simulink model "directMRACSystemModel"  (Simulink 7.3)
settings: Solver=ode45  StartTime=0.0  StopTime=tf  RelTol=1e-3
InitFcn:
  | initDirectMRACSystemModel
StopFcn:
  | plotlab
values from neighbouring files (symbols this model uses):
  Am = A - b*kx'    [initDirectMRACSystemMode_wPrj.m]    (also in initDirectMRACSystemModel.m; initDirectMRACSystemModel_wStatePred.m; initL1AdaptiveSystemModel.m)
  b = [0 ; d0]    [initDirectMRACSystemMode_wPrj.m]    (also in initDirectMRACSystemModel.m; initDirectMRACSystemModel_wStatePred.m; initL1AdaptiveSystemModel.m)
  c = [1 ; 1]    [initDirectMRACSystemMode_wPrj.m]    (also in initDirectMRACSystemModel.m; initDirectMRACSystemModel_wStatePred.m; initL1AdaptiveSystemModel.m)
  fx_p_absx1x2_1 = [theta(4) 0]    [initDirectMRACSystemMode_wPrj.m]    (also in initDirectMRACSystemModel.m; initDirectMRACSystemModel_wStatePred.m; initL1AdaptiveSystemModel.m)
  fx_p_absx1x2_2 = [theta(4) 0]    [initDirectMRACSystemMode_wPrj.m]    (also in initDirectMRACSystemModel.m; initDirectMRACSystemModel_wStatePred.m; initL1AdaptiveSystemModel.m)
  fx_p_absx2x2_1 = [theta(5) 0]    [initDirectMRACSystemMode_wPrj.m]    (also in initDirectMRACSystemModel.m; initDirectMRACSystemModel_wStatePred.m; initL1AdaptiveSystemModel.m)
  fx_p_absx2x2_2 = [theta(5) 0]    [initDirectMRACSystemMode_wPrj.m]    (also in initDirectMRACSystemModel.m; initDirectMRACSystemModel_wStatePred.m; initL1AdaptiveSystemModel.m)
  fx_p_x1_1 = [theta(6) 0 theta(2) theta(1)]    [initDirectMRACSystemMode_wPrj.m]    (also in initDirectMRACSystemModel.m; initDirectMRACSystemModel_wStatePred.m; initL1AdaptiveSystemModel.m)
  fx_p_x1_2 = [theta(6) 0 theta(2) theta(1)]    [initDirectMRACSystemMode_wPrj.m]    (also in initDirectMRACSystemModel.m; initDirectMRACSystemModel_wStatePred.m; initL1AdaptiveSystemModel.m)
  fx_p_x2_1 = [theta(3) 0]    [initDirectMRACSystemMode_wPrj.m]    (also in initDirectMRACSystemModel.m; initDirectMRACSystemModel_wStatePred.m; initL1AdaptiveSystemModel.m)
  fx_p_x2_2 = [theta(3) 0]    [initDirectMRACSystemMode_wPrj.m]    (also in initDirectMRACSystemModel.m; initDirectMRACSystemModel_wStatePred.m; initL1AdaptiveSystemModel.m)
  Gamma = 1*eye(2,2)    [initDirectMRACSystemModel.m]    (also in initDirectMRACSystemModel_wStatePred.m; initL1AdaptiveSystemModel.m = 20)
  kg = -(c'*(Am^-1)*b).^-1    [initDirectMRACSystemModel.m]    (also in initDirectMRACSystemModel_wStatePred.m; initL1AdaptiveSystemModel.m)
  kx = [0.25 ; 0.707]    [initDirectMRACSystemMode_wPrj.m]    (also in initDirectMRACSystemModel.m; initDirectMRACSystemModel_wStatePred.m; initL1AdaptiveSystemModel.m)
  kxtld0 = [200 200]'    [initDirectMRACSystemMode_wPrj.m]    (also in initDirectMRACSystemModel.m = zeros(2,1))
  P = lyap(Am',Q)    [initDirectMRACSystemMode_wPrj.m]    (also in initDirectMRACSystemModel.m; initDirectMRACSystemModel_wStatePred.m; initL1AdaptiveSystemModel.m)
  tNonlinChange = tNonlinEnable+10    (= 60)    [initDirectMRACSystemMode_wPrj.m]    (also in initDirectMRACSystemModel.m = 10; initDirectMRACSystemModel_wStatePred.m = 10; initL1AdaptiveSystemModel.m = 10)
  tNonlinEnable = 50    [initDirectMRACSystemMode_wPrj.m]    (also in initDirectMRACSystemModel.m = 0; initDirectMRACSystemModel_wStatePred.m = 0; initL1AdaptiveSystemModel.m = 0)
  x0 = zeros(2,1)    [initDirectMRACSystemMode_wPrj.m]    (also in initDirectMRACSystemModel.m; initDirectMRACSystemModel_wStatePred.m; initL1AdaptiveSystemModel.m)
  xm0 = zeros(2,1)    [initDirectMRACSystemMode_wPrj.m]    (also in initDirectMRACSystemModel.m)
libraries: dspmtrx3 x5, simulink x3
settings Model: Creator=alp.marangoz  LastModifiedBy=Alp
settings OptimizationCC: ExpressionDepthLimit=128
settings DebuggingCC: StateNameClashWarn=none  StrictBusMsg=ErrorLevel1
settings CodeAppCC: CustomSymbolStrType=$N$R$M_T
settings GRTTargetCC: CombineOutputUpdateFcns=on

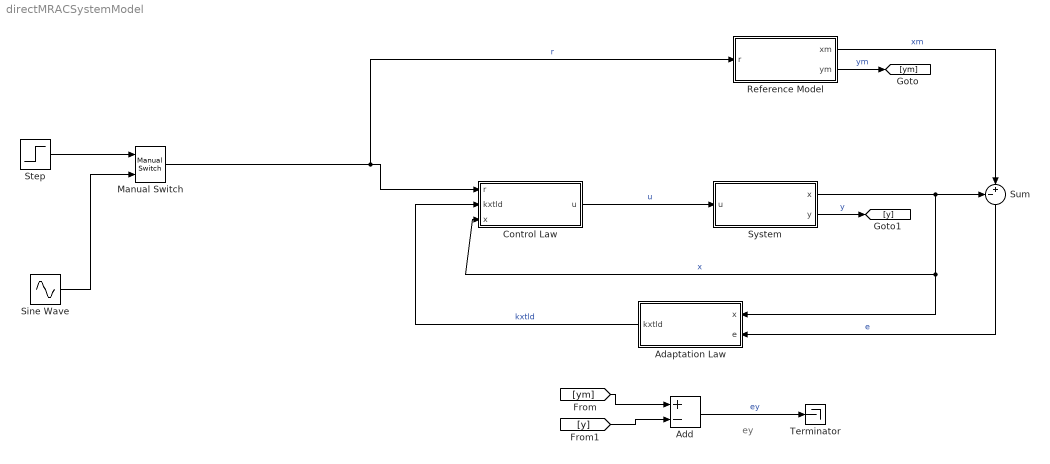
== system directMRACSystemModel ==
  note: ey
  Adaptation Law : Subsystem  TreatAsAtomicUnit=on
  Add : Sum  Inputs=+-  OutDataType=fixdt(1, 16)  OutScaling=2^-10
  Control Law : Subsystem  TreatAsAtomicUnit=on
  Manual Switch : simulink/Signal Routing/Manual Switch  SystemSampleTime=-1  sw=0  action=0  varsize=off
  Reference Model : Subsystem  TreatAsAtomicUnit=on
  Sine Wave : Sin  Amplitude=-2  Bias=0  Frequency=0.15  Phase=0  Samples=10  SampleTime=0  Offset=0
  Step : Step  SampleTime=0  VectorParams1D=off
  Sum : Sum  Inputs=-+|  OutDataType=fixdt(1, 16)  OutScaling=2^0
  System : Subsystem  TreatAsAtomicUnit=on
      settings: MinAlgLoopOccurrences=on
  Terminator : Terminator
  wires:
  Reference Model/1(xm) -> Sum/2  "xm"
  System/1(x) -> Sum/1, Adaptation Law/1(x), Control Law/3(x)  "x"
  Sum/1 -> Adaptation Law/2(e)  "e"
  Control Law/1(u) -> System/1(u)  "u"
  Adaptation Law/1(kxtld) -> Control Law/2(kxtld)  "kxtld"
  Manual Switch/1 -> Control Law/1(r), Reference Model/1(r)  "r"
  Reference Model/2(ym) -> [ym]  "ym"
  System/2(y) -> [y]  "y"
  [ym] -> Add/1
  [y] -> Add/2
  Add/1 -> Terminator/1  "ey"
  Step/1 -> Manual Switch/1
  Sine Wave/1 -> Manual Switch/2

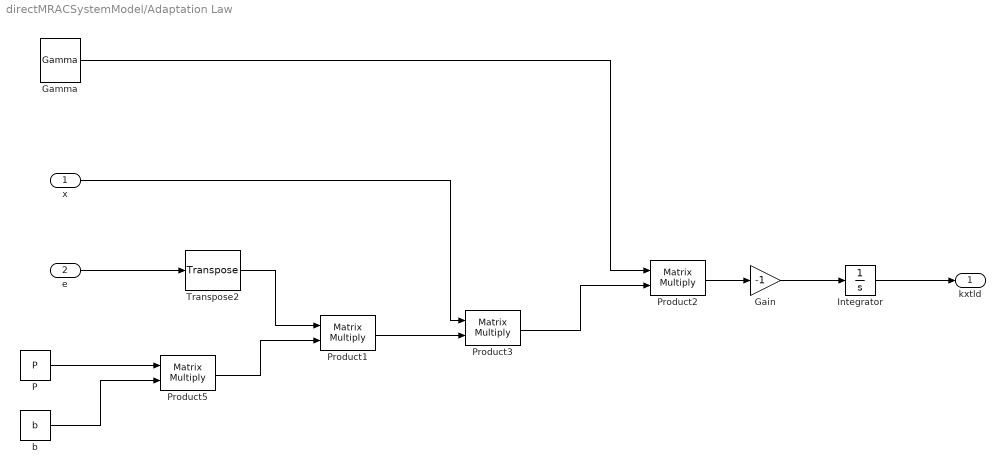
== system directMRACSystemModel/Adaptation Law ==
  x : Inport  OutDataType=fixdt(1, 16)  OutScaling=2^0
  e : Inport  Port=2  OutDataType=fixdt(1, 16)  OutScaling=2^0
  Gain : Gain  Gain=-1  ParameterDataType=fixdt(1, 16)  ParameterScaling=2^0  OutDataType=fixdt(1, 16)  OutScaling=2^0
  Gamma : Constant  Value=Gamma  VectorParams1D=off  OutDataType=fixdt(1, 16)  OutScaling=2^0
  Integrator : Integrator  InitialCondition=kxtld0
  P : Constant  Value=P  VectorParams1D=off  OutDataType=fixdt(1, 16)  OutScaling=2^0
  Product{1..3,5} (4 alike) : Product  Multiplication=Matrix(*)  OutDataType=fixdt(1, 16)  OutScaling=2^0  RndMeth=Zero
  Transpose2 : dspmtrx3/Transpose  SystemSampleTime=-1  Hermitian=off  overflowFlag=off
  b : Constant  Value=b  VectorParams1D=off  OutDataType=fixdt(1, 16)  OutScaling=2^0
  kxtld : Outport  OutDataType=fixdt(1, 16)  OutScaling=2^0
  wires:
  P/1 -> Product5/1
  b/1 -> Product5/2
  e/1 -> Transpose2/1
  Transpose2/1 -> Product1/1
  Product5/1 -> Product1/2
  x/1 -> Product3/1
  Product1/1 -> Product3/2
  Gamma/1 -> Product2/1
  Product3/1 -> Product2/2
  Product2/1 -> Gain/1
  Gain/1 -> Integrator/1
  Integrator/1 -> kxtld/1

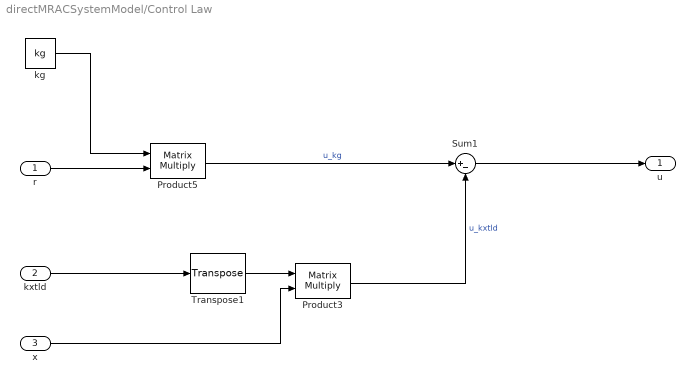
== system directMRACSystemModel/Control Law ==
  r : Inport  OutDataType=fixdt(1, 16)  OutScaling=2^0
  kxtld : Inport  Port=2  OutDataType=fixdt(1, 16)  OutScaling=2^0
  x : Inport  Port=3  OutDataType=fixdt(1, 16)  OutScaling=2^0
  Product3 : Product  Multiplication=Matrix(*)  OutDataType=fixdt(1, 16)  OutScaling=2^0  RndMeth=Zero
  Product5 : Product  Multiplication=Matrix(*)  OutDataType=fixdt(1, 16)  OutScaling=2^0  RndMeth=Zero
  Sum1 : Sum  Inputs=|+-  OutDataType=fixdt(1, 16)  OutScaling=2^0
  Transpose1 : dspmtrx3/Transpose  SystemSampleTime=-1  Hermitian=off  overflowFlag=off
  kg : Constant  Value=kg  VectorParams1D=off  OutDataType=fixdt(1, 16)  OutScaling=2^0
  u : Outport  OutDataType=fixdt(1, 16)  OutScaling=2^0
  wires:
  Transpose1/1 -> Product3/1
  kg/1 -> Product5/1
  r/1 -> Product5/2
  kxtld/1 -> Transpose1/1
  x/1 -> Product3/2
  Product5/1 -> Sum1/1  "u_kg"
  Product3/1 -> Sum1/2  "u_kxtld"
  Sum1/1 -> u/1

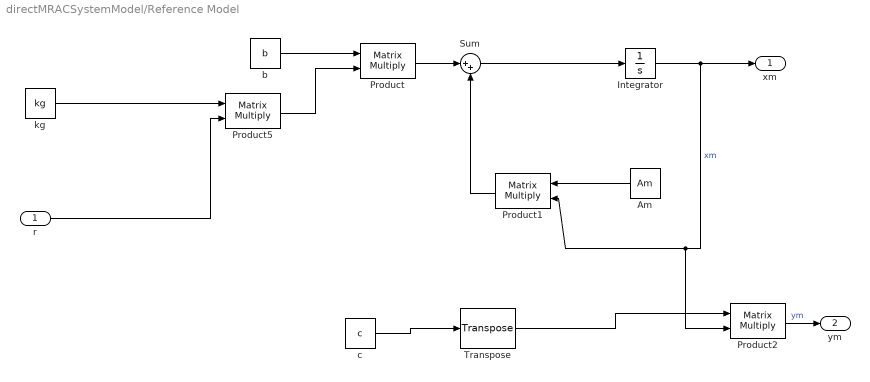
== system directMRACSystemModel/Reference Model ==
  r : Inport  OutDataType=fixdt(1, 16)  OutScaling=2^0
  Am : Constant  Value=Am  VectorParams1D=off  OutDataType=fixdt(1, 16)  OutScaling=2^0
  Integrator : Integrator  InitialCondition=xm0
  Product{,1..2,5} (4 alike) : Product  Multiplication=Matrix(*)  OutDataType=fixdt(1, 16)  OutScaling=2^0  RndMeth=Zero
  Sum : Sum  Inputs=|++  OutDataType=fixdt(1, 16)  OutScaling=2^0
  Transpose : dspmtrx3/Transpose  SystemSampleTime=-1  Hermitian=off  overflowFlag=off
  b : Constant  Value=b  VectorParams1D=off  OutDataType=fixdt(1, 16)  OutScaling=2^0
  c : Constant  Value=c  VectorParams1D=off  OutDataType=fixdt(1, 16)  OutScaling=2^0
  kg : Constant  Value=kg  VectorParams1D=off  OutDataType=fixdt(1, 16)  OutScaling=2^0
  xm : Outport  OutDataType=fixdt(1, 16)  OutScaling=2^0
  ym : Outport  Port=2  OutDataType=fixdt(1, 16)  OutScaling=2^0
  wires:
  c/1 -> Transpose/1
  Am/1 -> Product1/1
  Sum/1 -> Integrator/1
  Integrator/1 -> xm/1, Product1/2, Product2/2  "xm"
  Product1/1 -> Sum/2
  Product/1 -> Sum/1
  Transpose/1 -> Product2/1
  Product2/1 -> ym/1  "ym"
  b/1 -> Product/1
  Product5/1 -> Product/2
  kg/1 -> Product5/1
  r/1 -> Product5/2

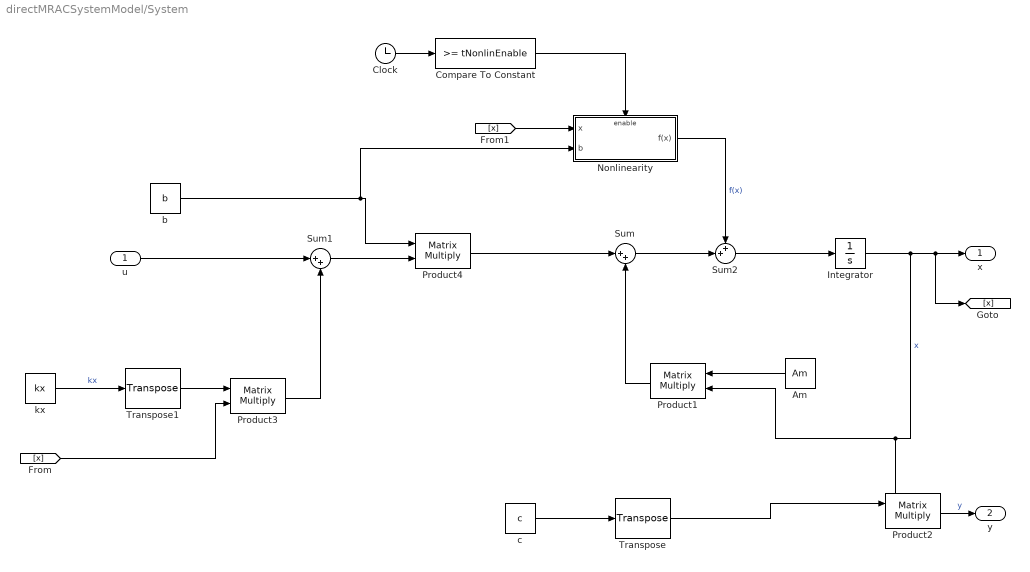
== system directMRACSystemModel/System ==
  u : Inport  OutDataType=fixdt(1, 16)  OutScaling=2^0
  Am : Constant  Value=Am  VectorParams1D=off  OutDataType=fixdt(1, 16)  OutScaling=2^0
  Clock : Clock
      settings: Decimation=10
  Compare To Constant : simulink/Logic and Bit Operations/Compare To Constant  SystemSampleTime=-1  relop=>=  const=tNonlinEnable  LogicOutDataTypeMode=uint8  ZeroCross=off
  Integrator : Integrator  InitialCondition=x0
  Nonlinearity : Subsystem  TreatAsAtomicUnit=on
  Product{1..4} (4 alike) : Product  Multiplication=Matrix(*)  OutDataType=fixdt(1, 16)  OutScaling=2^0  RndMeth=Zero
  Sum : Sum  Inputs=|++  OutDataType=fixdt(1, 16)  OutScaling=2^0
  Sum1 : Sum  Inputs=|++  OutDataType=fixdt(1, 16)  OutScaling=2^0
  Sum2 : Sum  Inputs=++|  OutDataType=fixdt(1, 16)  OutScaling=2^0
  Transpose : dspmtrx3/Transpose  SystemSampleTime=-1  Hermitian=off  overflowFlag=off
  Transpose1 : dspmtrx3/Transpose  SystemSampleTime=-1  Hermitian=off  overflowFlag=off
  b : Constant  Value=b  VectorParams1D=off  OutDataType=fixdt(1, 16)  OutScaling=2^0
  c : Constant  Value=c  VectorParams1D=off  OutDataType=fixdt(1, 16)  OutScaling=2^0
  kx : Constant  Value=kx  VectorParams1D=off  OutDataType=fixdt(1, 16)  OutScaling=2^0
  x : Outport  OutDataType=fixdt(1, 16)  OutScaling=2^0
  y : Outport  Port=2  OutDataType=fixdt(1, 16)  OutScaling=2^0
  wires:
  Product2/1 -> y/1  "y"
  Transpose/1 -> Product2/1
  Product1/1 -> Sum/2
  Integrator/1 -> Product2/2, Product1/2, x/1, [x]  "x"
  Am/1 -> Product1/1
  c/1 -> Transpose/1
  kx/1 -> Transpose1/1  "kx"
  Transpose1/1 -> Product3/1
  u/1 -> Sum1/1
  [x] -> Product3/2
  Product3/1 -> Sum1/2
  b/1 -> Product4/1, Nonlinearity/2(b)
  Sum1/1 -> Product4/2
  Product4/1 -> Sum/1
  Sum/1 -> Sum2/2
  [x] -> Nonlinearity/1(x)
  Sum2/1 -> Integrator/1
  Clock/1 -> Compare To Constant/1
  Compare To Constant/1 -> Nonlinearity/Enable
  Nonlinearity/1(f(x)) -> Sum2/1  "f(x)"

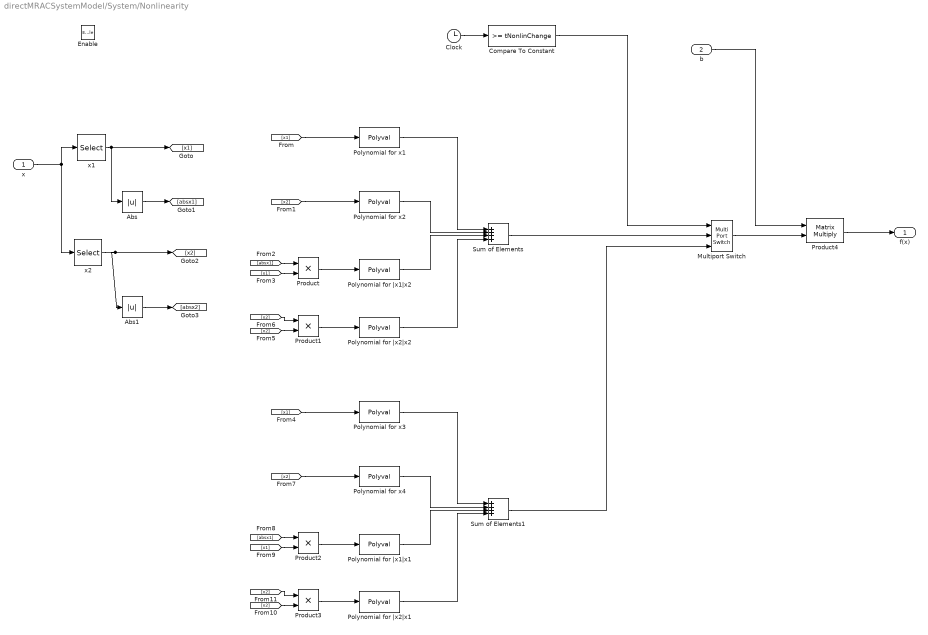
== system directMRACSystemModel/System/Nonlinearity ==
  x : Inport  OutDataType=fixdt(1, 16)  OutScaling=2^0
  b : Inport  Port=2  OutDataType=fixdt(1, 16)  OutScaling=2^0
  Enable : EnablePort
  Abs : Abs  OutDataType=fixdt(1, 16)  OutScaling=2^0
  Abs1 : Abs  OutDataType=fixdt(1, 16)  OutScaling=2^0
  Clock : Clock
      settings: Decimation=10
  Compare To Constant : simulink/Logic and Bit Operations/Compare To Constant  SystemSampleTime=-1  relop=>=  const=tNonlinChange  LogicOutDataTypeMode=uint8  ZeroCross=off
  Multiport Switch : MultiPortSwitch  Inputs=2  zeroidx=on  OutDataType=fixdt(1, 16)  OutScaling=2^0
  Polynomial for x1 : Polyval  Coefs=fx_p_x1_1
  Polynomial for x2 : Polyval  Coefs=fx_p_x2_1
  Polynomial for x3 : Polyval  Coefs=fx_p_x1_2
  Polynomial for x4 : Polyval  Coefs=fx_p_x2_2
  Polynomial for |x1|x1 : Polyval  Coefs=fx_p_absx1x2_2
  Polynomial for |x1|x2 : Polyval  Coefs=fx_p_absx1x2_1
  Polynomial for |x2|x1 : Polyval  Coefs=fx_p_absx2x2_2
  Polynomial for |x2|x2 : Polyval  Coefs=fx_p_absx2x2_1
  Product{,1..3} (4 alike) : Product  OutDataType=fixdt(1, 16)  OutScaling=2^0  RndMeth=Zero
  Product4 : Product  Multiplication=Matrix(*)  OutDataType=fixdt(1, 16)  OutScaling=2^0  RndMeth=Zero
  Sum of Elements : Sum  Inputs=++++  OutDataType=fixdt(1, 16)  OutScaling=2^-10
  Sum of Elements1 : Sum  Inputs=++++  OutDataType=fixdt(1, 16)  OutScaling=2^-10
  x1 : Selector  InputPortWidth=2  IndexOptions=Index vector (dialog)  Indices=[1 ]  OutputSizes=1
  x2 : Selector  InputPortWidth=2  IndexOptions=Index vector (dialog)  Indices=2  OutputSizes=1
  f(x) : Outport  OutDataType=fixdt(1, 16)  OutScaling=2^0
  wires:
  x/1 -> x2/1, x1/1
  x1/1 -> [x1], Abs/1
  Abs/1 -> [absx1]
  x2/1 -> [x2], Abs1/1
  Abs1/1 -> [absx2]
  Polynomial for x1/1 -> Sum of Elements/1
  Polynomial for x2/1 -> Sum of Elements/2
  Polynomial for |x1|x2/1 -> Sum of Elements/3
  Polynomial for |x2|x2/1 -> Sum of Elements/4
  [x1] -> Polynomial for x1/1
  [x2] -> Polynomial for x2/1
  [absx1] -> Product/1
  [x1] -> Product/2
  Product/1 -> Polynomial for |x1|x2/1
  [x2] -> Product1/1
  [x2] -> Product1/2
  Product1/1 -> Polynomial for |x2|x2/1
  Polynomial for x3/1 -> Sum of Elements1/1
  Polynomial for x4/1 -> Sum of Elements1/2
  Polynomial for |x1|x1/1 -> Sum of Elements1/3
  Polynomial for |x2|x1/1 -> Sum of Elements1/4
  [x1] -> Polynomial for x3/1
  [x2] -> Polynomial for x4/1
  [absx1] -> Product2/1
  [x1] -> Product2/2
  Product2/1 -> Polynomial for |x1|x1/1
  [x2] -> Product3/1
  [x2] -> Product3/2
  Product3/1 -> Polynomial for |x2|x1/1
  Clock/1 -> Compare To Constant/1
  Compare To Constant/1 -> Multiport Switch/1
  Sum of Elements/1 -> Multiport Switch/2
  Sum of Elements1/1 -> Multiport Switch/3
  b/1 -> Product4/1
  Multiport Switch/1 -> Product4/2
  Product4/1 -> f(x)/1
